simulink model "OpenLoopWindTurbineModel_withActuators2014"  (R2013b)
settings: Solver=ode4  SolverMode=SingleTasking  StartTime=0.0  StopTime=TIME_SIM  FixedStep=STEP_SIZE  MaxStep=Ts  RelTol=1e-6
undefined symbols (not defined in the file or in its folder): A, Bd, beta_max, beta_min, beta_OP, CP0, dbeta_max, dbeta_min, dgen_max, dgen_min, gen_max, gen_min, Jg, Jr, Kd, Lambda0, Ng, Pitch0, R, rho_air, tau_beta, tau_gen, Tg_OP, v_OP, x0
settings Model: Creator=roga  LastModifiedBy=roga
settings DataIOCC: SaveFinalState=on
settings DebuggingCC: StateNameClashWarn=warning

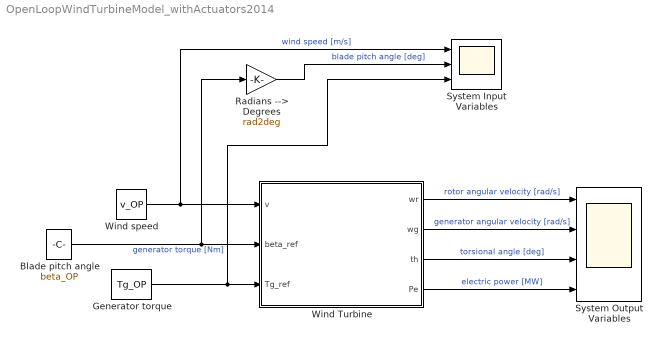
== system OpenLoopWindTurbineModel_withActuators2014 ==
  Blade pitch angle : Constant  Value=beta_OP
      mask Display: port_label('output',1,'\beta_{OP}','Interpreter','tex')
  Generator torque : Constant  Value=Tg_OP
      mask Display: port_label('output',1,'T_{g,OP}','Interpreter','tex')
  Radians --> Degrees : Gain  Gain=rad2deg
  System Input Variables : Scope  NumInputPorts=3
      settings: ShowLegends=on  YMin=-5~-5~-5  YMax=5~5~5
  System Output Variables : Scope  NumInputPorts=4
      settings: ShowLegends=on  YMin=-5~-5~-5~-5  YMax=5~5~5~5
  Wind Turbine : Subsystem
      mask Display:
      | image('wind_turbine.jpg')
      | port_label('input',1,'v')
      | port_label('input',2,'\beta_{ref}','Interpreter','tex')
      | port_label('input',3,'T_{g,ref}','Interpreter','tex')
      | port_label('output',1,'\omega_r','Interpreter','tex')
      | port_label('output',2,'\omega_g','Interpreter','tex')
      | port_label('output',3,'\theta','Interpreter','tex')
      | port_label('output',4,'P_e','Interpreter','tex')
  Wind speed : Constant  Value=v_OP
      mask Display: port_label('output',1,'v_{OP}','Interpreter','tex')
  wires:
  Wind speed/1 -> System Input Variables/1, Wind Turbine/1(v)  "wind speed [m/s]"
  Generator torque/1 -> System Input Variables/3, Wind Turbine/3(Tg_ref)  "generator torque [Nm]"
  Wind Turbine/1(wr) -> System Output Variables/1  "rotor angular velocity [rad/s]"
  Wind Turbine/2(wg) -> System Output Variables/2  "generator angular velocity [rad/s]"
  Wind Turbine/3(th) -> System Output Variables/3  "torsional angle [deg]"
  Wind Turbine/4(Pe) -> System Output Variables/4  "electric power [MW]"
  Radians --> Degrees/1 -> System Input Variables/2  "blade pitch angle [deg]"
  Blade pitch angle/1 -> Radians --> Degrees/1, Wind Turbine/2(beta_ref)

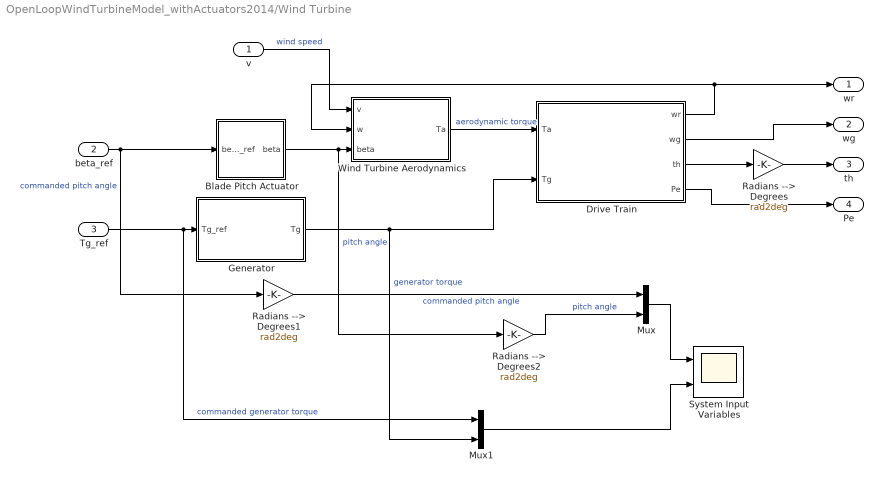
== system OpenLoopWindTurbineModel_withActuators2014/Wind Turbine ==
  v : Inport
  beta_ref : Inport  Port=2
  Tg_ref : Inport  Port=3
  Blade Pitch Actuator : Subsystem
      mask Display:
      | image('blades.jpg')
      | port_label('input',1,'\beta_{ref}','Interpreter','tex')
      | port_label('output',1,'\beta','Interpreter','tex')
  Drive Train : Subsystem
      mask Display:
      | image('wind_turbine_nacelle.jpg')
      | port_label('input',1,'T_a','Interpreter','tex')
      | port_label('input',2,'T_g','Interpreter','tex')
      | port_label('output',1,'\omega_r','Interpreter','tex')
      | port_label('output',2,'\omega_g','Interpreter','tex')
      | port_label('output',3,'\theta','Interpreter','tex')
      | port_label('output',4,'P_e','Interpreter','tex')
  Generator : Subsystem
      mask Display:
      | image('generator.jpg')
      | port_label('input',1,'T_{g,ref}','Interpreter','tex')
      | port_label('output',1,'T_g','Interpreter','tex')
  Mux : Mux  Inputs=2
  Mux1 : Mux  Inputs=2
  Radians --> Degrees : Gain  Gain=rad2deg
  Radians --> Degrees1 : Gain  Gain=rad2deg
  Radians --> Degrees2 : Gain  Gain=rad2deg
  System Input Variables : Scope  NumInputPorts=2
      settings: ShowLegends=on  YMin=0~40680.3  YMax=1050~40680.3  SaveName=ScopeData2
  Wind Turbine Aerodynamics : Subsystem
      mask Display:
      | image('PowerCoefficient.jpg')
      | port_label('input',1,'v')
      | port_label('input',2,'\omega_r','Interpreter','tex')
      | port_label('input',3,'\beta','Interpreter','tex')
      | port_label('output',1,'T_a','Interpreter','tex')
  wr : Outport
  wg : Outport  Port=2
  th : Outport  Port=3
  Pe : Outport  Port=4
  wires:
  Drive Train/1(wr) -> wr/1, Wind Turbine Aerodynamics/2(w)
  Drive Train/2(wg) -> wg/1
  Drive Train/3(th) -> Radians --> Degrees/1
  Drive Train/4(Pe) -> Pe/1
  Wind Turbine Aerodynamics/1(Ta) -> Drive Train/1(Ta)  "aerodynamic torque"
  Radians --> Degrees/1 -> th/1
  v/1 -> Wind Turbine Aerodynamics/1(v)  "wind speed"
  beta_ref/1 -> Radians --> Degrees1/1, Blade Pitch Actuator/1(beta_ref)  "commanded pitch angle"
  Blade Pitch Actuator/1(beta) -> Radians --> Degrees2/1, Wind Turbine Aerodynamics/3(beta)  "pitch angle"
  Generator/1(Tg) -> Mux1/2, Drive Train/2(Tg)  "generator torque"
  Tg_ref/1 -> Mux1/1, Generator/1(Tg_ref)  "commanded generator torque"
  Mux/1 -> System Input Variables/1
  Mux1/1 -> System Input Variables/2
  Radians --> Degrees1/1 -> Mux/1  "commanded pitch angle"
  Radians --> Degrees2/1 -> Mux/2  "pitch angle"

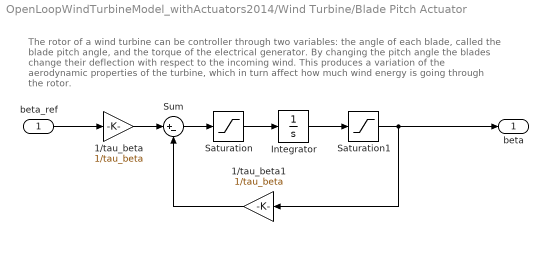
== system OpenLoopWindTurbineModel_withActuators2014/Wind Turbine/Blade Pitch Actuator ==
  note: The rotor of a wind turbine can be controller through two variables: the angle of each blade,
      | called the blade pitch angle, and the torque of the electrical generator. By changing the pitch
      | angle the blades change their deflection with respect to the incoming wind. This produces a
      | variation of the aerodynamic properties of the turbine, which in turn affect how much wind energy
      | is going through the rotor.
  beta_ref : Inport
  1/tau_beta : Gain  Gain=1/tau_beta
  1/tau_beta1 : Gain  Gain=1/tau_beta
  Integrator : Integrator  Priority=4  InitialCondition=x0(4)
  Saturation : Saturate  UpperLimit=dbeta_max  LowerLimit=dbeta_min
  Saturation1 : Saturate  UpperLimit=beta_max  LowerLimit=beta_min
  Sum : Sum  Inputs=|+-
  beta : Outport
  wires:
  Saturation/1 -> Integrator/1
  1/tau_beta/1 -> Sum/1
  beta_ref/1 -> 1/tau_beta/1
  1/tau_beta1/1 -> Sum/2
  Integrator/1 -> Saturation1/1
  Sum/1 -> Saturation/1
  Saturation1/1 -> beta/1, 1/tau_beta1/1

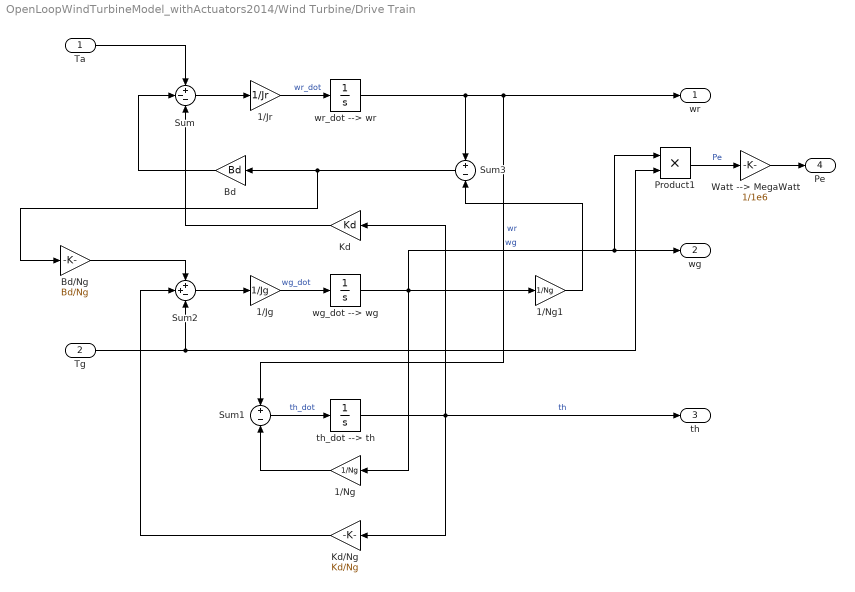
== system OpenLoopWindTurbineModel_withActuators2014/Wind Turbine/Drive Train ==
  Ta : Inport
  Tg : Inport  Port=2
  1/Jg : Gain  Gain=1/Jg
  1/Jr : Gain  Gain=1/Jr
  1/Ng : Gain  Gain=1/Ng
  1/Ng1 : Gain  Gain=1/Ng
  Bd : Gain  Gain=Bd
  Bd/Ng : Gain  Gain=Bd/Ng
  Kd : Gain  Gain=Kd
  Kd/Ng : Gain  Gain=Kd/Ng
  Product1 : Product
  Sum : Sum  Inputs=+--
  Sum1 : Sum  Inputs=+-
  Sum2 : Sum  Inputs=++-
  Sum3 : Sum  Inputs=+-
  Watt --> MegaWatt : Gain  Gain=1/1e6
  th_dot --> th : Integrator  Priority=3  InitialCondition=x0(3)  LowerSaturationLimit=0
  wg_dot --> wg : Integrator  Priority=2  InitialCondition=x0(2)  LowerSaturationLimit=0
  wr_dot --> wr : Integrator  Priority=1  InitialCondition=x0(1)  LowerSaturationLimit=0
  wr : Outport
  wg : Outport  Port=2
  th : Outport  Port=3
  Pe : Outport  Port=4
  wires:
  wg_dot --> wg/1 -> Product1/1, wg/1, 1/Ng1/1, 1/Ng/1  "wg"
  wr_dot --> wr/1 -> Sum3/1, wr/1, Sum1/1  "wr"
  1/Ng/1 -> Sum1/2
  Sum1/1 -> th_dot --> th/1  "th_dot"
  Sum2/1 -> 1/Jg/1
  1/Ng1/1 -> Sum3/2
  Sum/1 -> 1/Jr/1
  1/Jr/1 -> wr_dot --> wr/1  "wr_dot"
  th_dot --> th/1 -> th/1, Kd/Ng/1, Kd/1  "th"
  1/Jg/1 -> wg_dot --> wg/1  "wg_dot"
  Sum3/1 -> Bd/Ng/1, Bd/1
  Bd/1 -> Sum/2
  Kd/1 -> Sum/3
  Bd/Ng/1 -> Sum2/1
  Kd/Ng/1 -> Sum2/2
  Ta/1 -> Sum/1
  Tg/1 -> Product1/2, Sum2/3
  Product1/1 -> Watt --> MegaWatt/1  "Pe"
  Watt --> MegaWatt/1 -> Pe/1

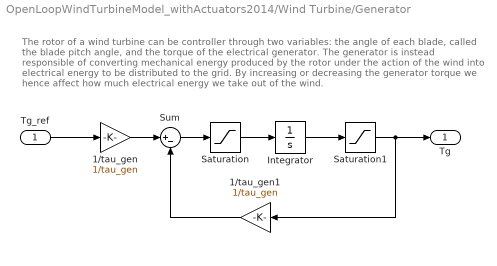
== system OpenLoopWindTurbineModel_withActuators2014/Wind Turbine/Generator ==
  note: The rotor of a wind turbine can be controller through two variables: the angle of each blade,
      | called the blade pitch angle, and the torque of the electrical generator. The generator is instead
      | responsible of converting mechanical energy produced by the rotor under the action of the wind
      | into electrical energy to be distributed to the grid. By increasing or decreasing the generator
      | torque we hence affect how much electrical energy we take out of the wind.
  Tg_ref : Inport
  1/tau_gen : Gain  Gain=1/tau_gen
  1/tau_gen1 : Gain  Gain=1/tau_gen
  Integrator : Integrator  Priority=5  InitialCondition=x0(5)
  Saturation : Saturate  UpperLimit=dgen_max  LowerLimit=dgen_min
  Saturation1 : Saturate  UpperLimit=gen_max  LowerLimit=gen_min
  Sum : Sum  Inputs=|+-
  Tg : Outport
  wires:
  Saturation1/1 -> Tg/1, 1/tau_gen1/1
  Sum/1 -> Saturation/1
  Integrator/1 -> Saturation1/1
  1/tau_gen1/1 -> Sum/2
  Tg_ref/1 -> 1/tau_gen/1
  1/tau_gen/1 -> Sum/1
  Saturation/1 -> Integrator/1

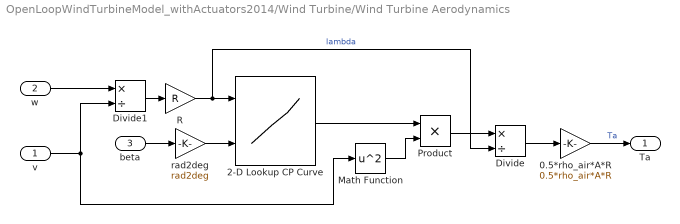
== system OpenLoopWindTurbineModel_withActuators2014/Wind Turbine/Wind Turbine Aerodynamics ==
  v : Inport
  w : Inport  Port=2
  beta : Inport  Port=3
  0.5*rho_air*A*R : Gain  Gain=0.5*rho_air*A*R
  2-D Lookup CP Curve : Lookup_n-D  BreakpointsForDimension1=Lambda0  BreakpointsForDimension2=Pitch0  BreakpointsForDimension3=CP0'  Table=CP0  DiagnosticForOutOfRangeInput=Warning  RndMeth=Simplest  InputSameDT=on
  Divide : Product  Inputs=*/
  Divide1 : Product  Inputs=*/
  Math Function : Math  Operator=square  SaturateOnIntegerOverflow=on
  Product : Product
  R : Gain  Gain=R
  rad2deg : Gain  Gain=rad2deg
  Ta : Outport
  wires:
  0.5*rho_air*A*R/1 -> Ta/1  "Ta"
  beta/1 -> rad2deg/1
  w/1 -> Divide1/1
  Divide/1 -> 0.5*rho_air*A*R/1
  Product/1 -> Divide/1
  Math Function/1 -> Product/2
  2-D Lookup CP Curve/1 -> Product/1
  v/1 -> Divide1/2, Math Function/1
  Divide1/1 -> R/1
  R/1 -> Divide/2, 2-D Lookup CP Curve/1  "lambda"
  rad2deg/1 -> 2-D Lookup CP Curve/2
